simulink model "modello_la_gs"  (R2023a)
settings: Solver=VariableStepAuto  StartTime=0.0  StopTime=20  RelTol=1e-3
values from neighbouring files (symbols this model uses):
  K_S = [K_S; K]    [LA.m]
  parametri = [V_1, L, d, alpha, beta]    [LA.m]
  u_eq_S = [u_eq_S u_eq_0]    [LA.m]
  x_0 = [0; 0; 0]    [LA.m]
  x_eq_S = [x_eq_S x_eq_0]    [LA.m]
undefined symbols (not defined in the file or in its folder): sigbuilder_block
settings Model: Creator=Randy  LastModifiedBy=Randy

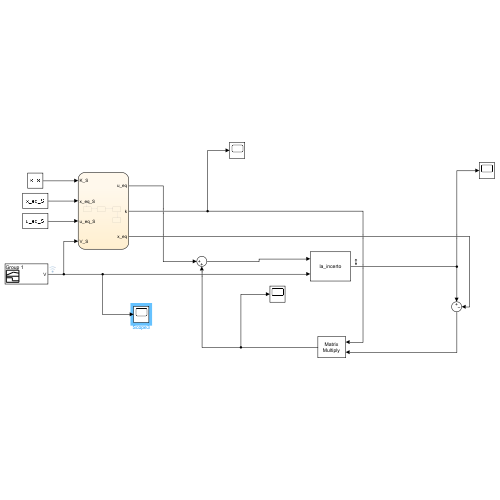
[thumbnail: Simulink's stored preview of the top-level diagram]
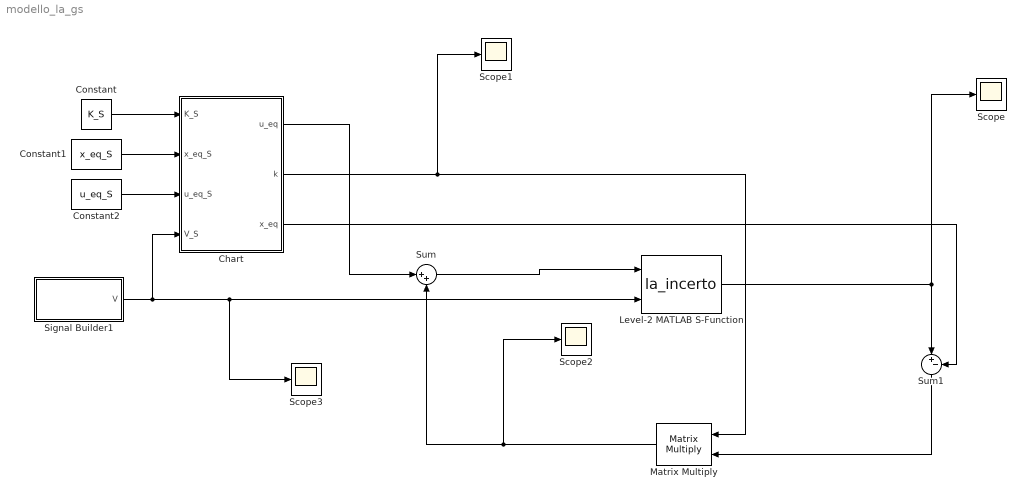
== system modello_la_gs ==
  Chart : Stateflow chart  TreatAsAtomicUnit=on
  Constant : Constant  Value=K_S
  Constant1 : Constant  Value=x_eq_S
  Constant2 : Constant  Value=u_eq_S
  Level-2 MATLAB S-Function : M-S-Function  FunctionName=la_incerto  Parameters=x_0,parametri
  Matrix Multiply : Product  Multiplication=Matrix(*)
  Scope{,1..3} (4 alike) : Scope
  Signal Builder1 : Subsystem  Tag=STV Subsys  LoadFcn=sigbuilder_block('load');  StartFcn=sigbuilder_block('start');  StopFcn=sigbuilder_block('stop');  ClipboardFcn=sigbuilder_block('clipboard');  mask(Sigbuilder block){tuvar=[0:10]}
      mask help: Simulink:masks:SigbuilderBlock_MD
      mask init:
      | if ~strcmp(get_param(bdroot(gcbh),'SimulationStatus'),'stopped') tuvar = sigbuilder_block('maskInit'); end
      settings: CopyFcn=sigbuilder_block('copy');  DeleteFcn=sigbuilder_block('delete');  ModelCloseFcn=sigbuilder_block('modelClose');  PreSaveFcn=sigbuilder_block('preSave');  PauseFcn=sigbuilder_block('pause');  ContinueFcn=sigbuilder_block('continue');  NameChangeFcn=sigbuilder_block('namechange');  OpenFcn=sigbuilder_block('open',[6 30 1012.5 470.25 ]);  CloseFcn=sigbuilder_block('close');
      mask Display: plot(0, 0, 100, 100,[2, 2, 32, 32, 2], [68, 8, 8, 68, 68],[32, 2], [38, 38], [32, 19, 2],[53, 60, 44], [32, 17, 17, 2],[16, 16, 31, 31]);txt = getActiveGroup(gcbh);text(2, 100, txt,'verticalAlignment', 'top');
  Sum : Sum  Inputs=|++
  Sum1 : Sum  Inputs=|+-
  wires:
  Chart/2(k) -> Scope1/1, Matrix Multiply/1
  Constant/1 -> Chart/1(K_S)
  Matrix Multiply/1 -> Scope2/1, Sum/2
  Sum1/1 -> Matrix Multiply/2
  Signal Builder1/1(V) -> Chart/4(V_S), Scope3/1, Level-2 MATLAB S-Function/2
  Chart/1(u_eq) -> Sum/1
  Constant2/1 -> Chart/3(u_eq_S)
  Constant1/1 -> Chart/2(x_eq_S)
  Sum/1 -> Level-2 MATLAB S-Function/1
  Level-2 MATLAB S-Function/1 -> Scope/1, Sum1/1
  Chart/3(x_eq) -> Sum1/2

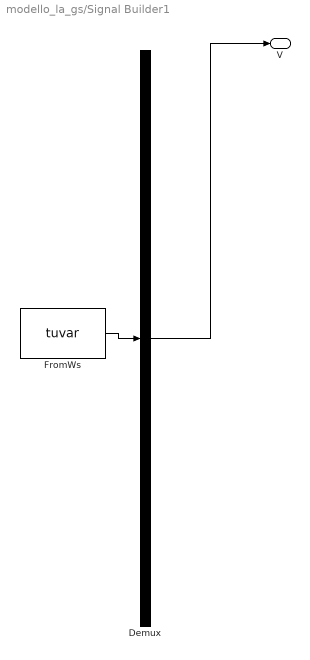
== system modello_la_gs/Signal Builder1 ==
  Demux : Demux  Tag=STV Demux  Outputs=1
      settings: DisplayOption=none
  FromWs : FromWorkspace  Tag=STV FromWs  VariableName=tuvar
      SigBuilderData=|
      | common.afterFinalStr = 'Extrapolate'
      | common.sampleTime = 0
      | dataSet.timeRange = [0 20]
      | dataSet.name = 'Group 1'
      | sbobj.Groups.Name = 'Group 1'
      | sbobj.Groups.Signals.Name = 'V'
      | sbobj.Groups.Signals.XData = [0 5 5 10 10 15 15 20]
      | sbobj.Groups.Signals.YData = [90 90 110 110 130 130 150 150]
      | sbobj.Groups.TimeRange = [0 20]
  V : Outport  Tag=STV Outport  VectorParamsAs1DForOutWhenUnconnected=off
  wires:
  Demux/1 -> V/1
  FromWs/1 -> Demux/1

== stateflow chart modello_la_gs/Chart ==
  state S0
    entry:
    x_eq = x_eq_S(1:3,1);
    u_eq = u_eq_S(1,1:1);
    k = K_S(1:1,1:3);
  state S1
    entry:
    x_eq = x_eq_S(1:3,2);
    u_eq = u_eq_S(1,1:1);
    k = K_S(2:2,1:3);
  state S2
    entry:
    x_eq = x_eq_S(1:3,3);
    u_eq = u_eq_S(1,1:1);
    k = K_S(3:3,1:3);
  state S3
    entry:
    x_eq = x_eq_S(1:3,4);
    u_eq = u_eq_S(1,1:1);
    k = K_S(4:4,1:3);
  (default) -> S0 : {V_S == 90}
  S1 -> S2 : [V_S == 130]
  S0 -> S1 : [V_S == 110]
  S2 -> S3 : [V_S == 150]
  data: K_S input; x_eq_S input; u_eq_S input; u_eq output; k output; x_eq output; V_S input
